simulink model "joy_controller"  (R2019b)
settings: Solver=VariableStepAuto  StartTime=0.0  StopTime=10.0  RelTol=1e-3
undefined symbols (not defined in the file): Axes, Buttons
libraries: robotlib x7
settings Model: Creator=oak  LastModifiedBy=oak

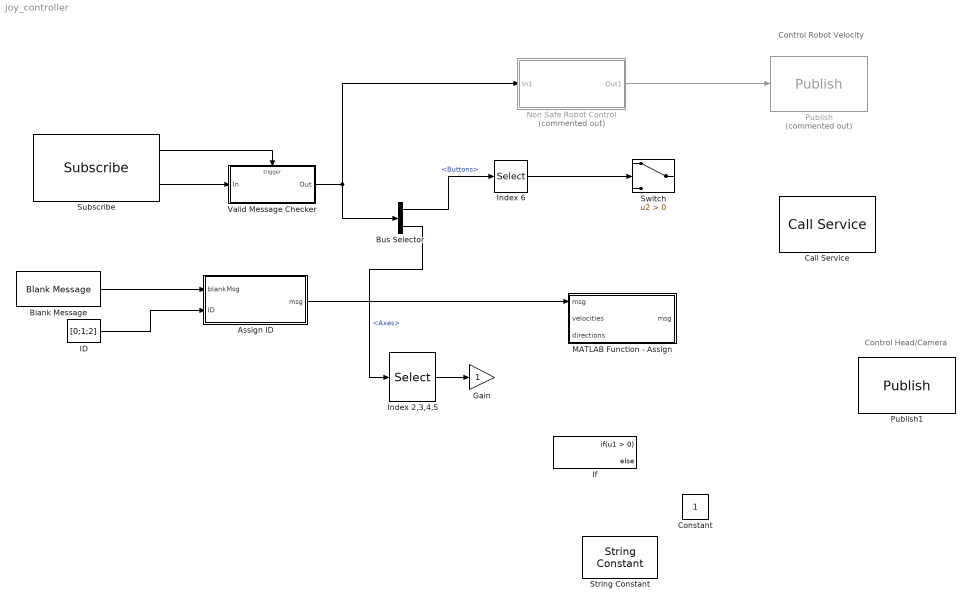
== system joy_controller ==
  note: Control Head/Camera
  note: Control Robot Velocity
  Assign ID : MATLAB Function  TreatAsAtomicUnit=on
  Blank Message : robotlib/Blank Message  messageClass=Message  entityType=sensor_msgs/JointState  messageType=sensor_msgs/JointState  SampleTime=inf
      settings: SourceProductName=ROS Toolbox
  Bus Selector : BusSelector  OutputSignals=Buttons,Axes
  Call Service : robotlib/Call Service  topicSource=Select from ROS network  service=/display/lift  serviceType=std_srvs/SetBool  connectionTimeout=5  keepPersistent=off  ShowErrorCodeOutput=on
      settings: SourceProductName=ROS Toolbox  SourceProductBaseCode=RR
  Constant : Constant
  Gain : Gain
  ID : Constant  Value=[0;1;2]
  If : If
  Index 2,3,4,5 : Selector  InputPortWidth=8  IndexOptions=Index vector (dialog)  Indices=[2,3,4,5]  OutputSizes=1
  Index 6 : Selector  IndexMode=Zero-based  InputPortWidth=11  IndexOptions=Index vector (dialog)  Indices=[6]  OutputSizes=1
  MATLAB Function - Assign : MATLAB Function  TreatAsAtomicUnit=on
  Non Safe Robot Control : Subsystem  Commented=on
  Publish : robotlib/Publish  Commented=on  topicSource=Specify your own  topic=/cmd_vel  messageType=geometry_msgs/Twist  messageQueueLength=1
      settings: SourceProductName=ROS Toolbox
  Publish1 : robotlib/Publish  topicSource=Select from ROS network  topic=/head/target_position  messageType=sensor_msgs/JointState  messageQueueLength=1
      settings: SourceProductName=ROS Toolbox
  String Constant : StringConstant
  Subscribe : robotlib/Subscribe  topicSource=Select from ROS network  topic=/joy  messageType=sensor_msgs/Joy  sampleTime=15  messageQueueLength=1
      settings: SourceProductName=ROS Toolbox
  Switch : Switch  Criteria=u2 > Threshold
  Valid Message Checker : Subsystem  TreatAsAtomicUnit=on
  wires:
  Valid Message Checker/1("Out ") -> Non Safe Robot Control/1(In1), Bus Selector/1
  Subscribe/1 -> Valid Message Checker/Trigger
  Subscribe/2 -> Valid Message Checker/1("In ")
  Non Safe Robot Control/1(Out1) -> Publish/1
  Blank Message/1 -> Assign ID/1(blankMsg)
  Assign ID/1(msg) -> MATLAB Function - Assign/1("msg ")
  ID/1 -> Assign ID/2(ID)
  Bus Selector/1 -> Index 6/1  "<Buttons>"
  Bus Selector/2 -> Index 2,3,4,5/1  "<Axes>"
  Index 6/1 -> Switch/2
  Index 2,3,4,5/1 -> Gain/1

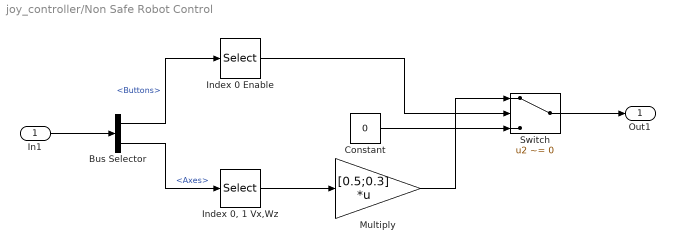
== system joy_controller/Non Safe Robot Control ==
  In1 : Inport
  Bus Selector : BusSelector  OutputSignals=Buttons,Axes
  Constant : Constant  Value=0
  Index 0 Enable : Selector  IndexMode=Zero-based  InputPortWidth=11  IndexOptions=Index vector (dialog)  Indices=[0]  OutputSizes=1
  "Index 0, 1 Vx,Wz" : Selector  IndexMode=Zero-based  InputPortWidth=8  IndexOptions=Index vector (dialog)  Indices=[0 1]  OutputSizes=1
  Multiply : Gain  Gain=[0.5;0.3]  Multiplication=Matrix(K*u)
  Switch : Switch  Criteria=u2 ~= 0
  Out1 : Outport
  wires:
  "Index 0, 1 Vx,Wz"/1 -> Multiply/1
  Index 0 Enable/1 -> Switch/2
  Multiply/1 -> Switch/1
  Bus Selector/1 -> Index 0 Enable/1  "<Buttons>"
  In1/1 -> Bus Selector/1
  Constant/1 -> Switch/3
  Switch/1 -> Out1/1
  Bus Selector/2 -> "Index 0, 1 Vx,Wz"/1  "<Axes>"

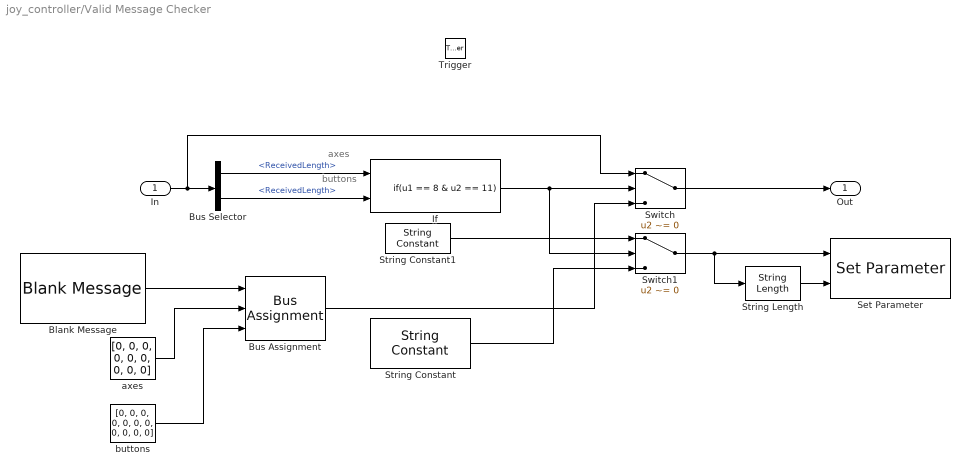
== system joy_controller/Valid Message Checker ==
  note: axes
  note: buttons
  "In " : Inport
  Trigger : TriggerPort  VariantControl=Variant
  Blank Message : robotlib/Blank Message  messageClass=Message  entityType=sensor_msgs/Joy  messageType=sensor_msgs/Joy  SampleTime=inf
      settings: SourceProductName=ROS Toolbox
  Bus Assignment : BusAssignment  AssignedSignals=Axes,Buttons
  Bus Selector : BusSelector  OutputSignals=Axes_SL_Info.ReceivedLength,Buttons_SL_Info.ReceivedLength
  If : If  NumInputs=2  IfExpression=u1 == 8 & u2 == 11  ShowElse=off
  Set Parameter : robotlib/Set Parameter  ParameterSource=Specify your own  ParameterName=/fault/joy  ParameterType=uint8[] (string)  ModelName=joy_controller  BlockId=ParamSet_joy_controller_32
      settings: SourceProductName=ROS Toolbox  SourceProductBaseCode=RR
  String Constant : StringConstant  String='JOY_SPEC_ERROR'
  String Constant1 : StringConstant  String=''
  String Length : StringLength
  Switch : Switch  Criteria=u2 ~= 0
  Switch1 : Switch  Criteria=u2 ~= 0
  axes : Constant  Value=[0, 0, 0, 0, 0, 0, 0, 0, 0]
  buttons : Constant  Value=[0, 0, 0, 0, 0, 0, 0, 0, 0, 0, 0]
  "Out " : Outport
  wires:
  "In "/1 -> Switch/1, Bus Selector/1
  Bus Selector/1 -> If/1  "<ReceivedLength>"
  Bus Selector/2 -> If/2  "<ReceivedLength>"
  If/1 -> Switch1/2, Switch/2
  Switch/1 -> "Out "/1
  String Constant/1 -> Switch1/3
  String Constant1/1 -> Switch1/1
  String Length/1 -> Set Parameter/2
  Switch1/1 -> String Length/1, Set Parameter/1
  Blank Message/1 -> Bus Assignment/1
  buttons/1 -> Bus Assignment/3
  axes/1 -> Bus Assignment/2
  Bus Assignment/1 -> Switch/3

== matlab function joy_controller/MATLAB Function - Assign ==
  data: msg input; velocities input; msg output; directions input
function msg = assignArrayValues(msg, velocities, directions)
%#codegen

% To set datatype of MSG output:
%  1. Create buses for this model: robotics.ros.createSimulinkBus(gcs)
%  1. Click "Edit Data" in  Toolstrip to open "Ports and Data Manager"
%  2. Select MSG and set datatype to "Bus: SL_Bus_<modelname>_<messageType>"
% See: 
% http://www.mathworks.com/help/simulink/ug/create-structures-in-matlab-function-blocks.html

% blankMessage (sensor_msgs/LaserScan) consists of 
%             Header: [1x1 Header]
%           AngleMin: 0
%           AngleMax: 0
%     AngleIncrement: 0
%      TimeIncrement: 0
%           ScanTime: 0
%           RangeMin: 0
%           RangeMax: 0
%             Ranges: [0x1 single]
%        Intensities: [0x1 single]

% Set Ranges array to have length 10, and modify indices 1, 3, 5 and 10
blankMessage.Ranges_SL_Info.CurrentLength = uint32(10); 
blankMessage.Ranges([1 3 5 7]) = velocities + [1 2 3 4];

msg = blankMessage;

== matlab function joy_controller/Assign ID ==
  data: blankMsg input; msg output Bus: SL_Bus_robotROSMessageUsageExample_sensor_msgs_JointState; ID input
function msg = stringArrayAssignID(blankMsg, ID)
% stringArrayAssign - Assign a string array in a ROS message
%
%  blankMsg (input): A bus for a 'sensor_msgs/JointState' message. This is 
%      used to initialize the output.
%  msg (output): A bus for a 'sensor_msgs/JointState' message message, with 
%      Name field set to a string array.
%
%   Copyright 2015 The MathWorks, Inc.

%#codegen

% Note: The datatype of 'msg' has been explicitly set to the appropriate 
% Simulink bus type ("SL_Bus_robotROSMessageUsageExample_sensor_msgs_JointState"). 
%
% If the model name is changed, the datatype needs to be changed as well:
%   1) Click "Edit Data" in the Editor toolstrip to open "Ports and Data Manager"
%   2) Select "msg". From the "Type" dropdown, select "--- Refresh data types ---"
%   3) Set datatype to "Bus: SL_Bus_<modelname>_sensor_msgs_JointState"

strArrayToAssign = {ID(0), ID(1), ID(2)};
msg = blankMsg;

% Set the number of strings in the string array.
% msg (sensor_msgs/JointState) includes the following fields
%           Name : array of std_msgs/String (string array)
%   Name_SL_Info : struct with fields CurrentLength, ReceivedLength
numStringsInArray = length(strArrayToAssign);
msg.Name_SL_Info.CurrentLength = uint32(numStringsInArray);

% Set the individual strings in the array
for idx=1:numStringsInArray
    str = strArrayToAssign{idx};
    strLength = length(str);
    msg.Name(idx).Data(1:strLength) = uint8(str);
    msg.Name(idx).Data_SL_Info.CurrentLength = uint32(strLength);
end
